simulink model "VelocityProfileStraightPath"  (R2019b)
settings: Solver=VariableStepAuto  StartTime=0.0  StopTime=10.0  RelTol=1e-3
libraries: drivinglib x1
settings Model: Creator=The MathWorks, Inc.  LastModifiedBy=varad
settings DataIOCC: SaveFormat=Structure
settings DebuggingCC: SymbolicDimsDataTypeCodeGenerationDiagnostic=none
settings SFSimCC: CustomCodeUndefinedFunction=UseInterfaceOnly

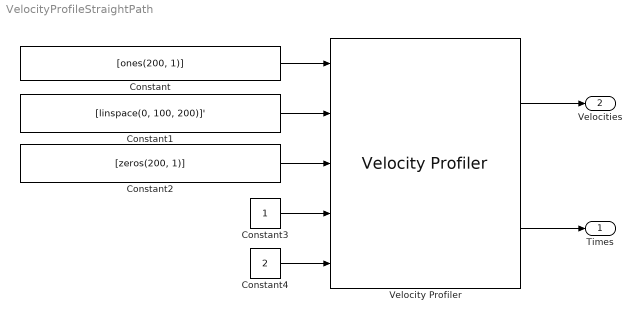
== system VelocityProfileStraightPath ==
  Constant : Constant  Value=[ones(200, 1)]
  Constant1 : Constant  Value=[linspace(0, 100, 200)]'
  Constant2 : Constant  Value=[zeros(200, 1)]
  Constant3 : Constant
  Constant4 : Constant  Value=2
  Velocity Profiler : drivinglib/Velocity Profiler  MaxLongitudinalAccel=3  MaxLongitudinalDecel=6  MaxSpeed=10  MaxLongitudinalJerk=1  MaxLateralAccel=1  ShowOptionalOutport=on  SampleTime=0.1  SimulateUsing=Code generation
      settings: SourceProductName=Automated Driving Toolbox  SourceProductBaseCode=DR
  Times : Outport  VectorParamsAs1DForOutWhenUnconnected=off
  Velocities : Outport  Port=2  VectorParamsAs1DForOutWhenUnconnected=off
  wires:
  Constant/1 -> Velocity Profiler/1
  Constant1/1 -> Velocity Profiler/2
  Constant2/1 -> Velocity Profiler/3
  Constant3/1 -> Velocity Profiler/4
  Constant4/1 -> Velocity Profiler/5
  Velocity Profiler/2 -> Times/1
  Velocity Profiler/1 -> Velocities/1
